simulink model "dcmotor"  (R2023b)
settings: Solver=VariableStepAuto  StartTime=0.0  StopTime=10  RelTol=10e-6
undefined symbols (not defined in the file): B, J, Ke, Ki, Kp, Kt, La, Ra, TL
settings Model: Creator=FM22  LastModifiedBy=FM22

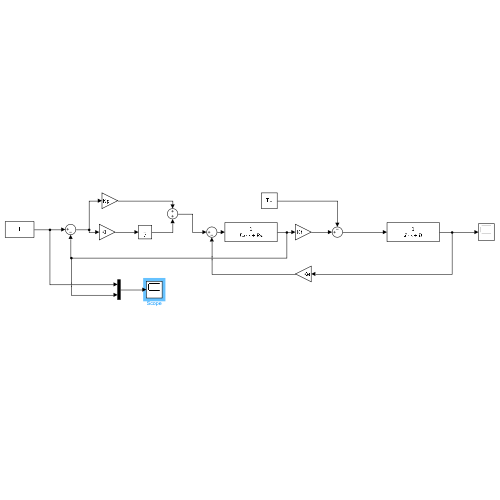
[thumbnail: Simulink's stored preview of the top-level diagram]
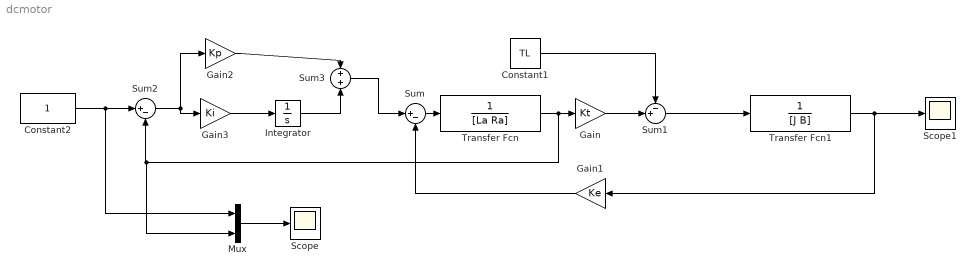
== system dcmotor ==
  Constant1 : Constant  Value=TL
  Constant2 : Constant
  Gain : Gain  Gain=Kt
  Gain1 : Gain  Gain=Ke
  Gain2 : Gain  Gain=Kp
  Gain3 : Gain  Gain=Ki
  Integrator : Integrator
  Mux : Mux  Inputs=2
  Scope : Scope
  Scope1 : Scope
  Sum : Sum  Inputs=|+-
  Sum1 : Sum  Inputs=-+|
  Sum2 : Sum  Inputs=|+-
  Sum3 : Sum  Inputs=+|+
  Transfer Fcn : TransferFcn  Denominator=[La Ra]
  Transfer Fcn1 : TransferFcn  Denominator=[J B]  ParameterTunability=Unconstrained
  wires:
  Sum/1 -> Transfer Fcn/1
  Transfer Fcn/1 -> Mux/2, Sum2/2, Gain/1
  Gain/1 -> Sum1/2
  Constant1/1 -> Sum1/1
  Sum1/1 -> Transfer Fcn1/1
  Gain1/1 -> Sum/2
  Transfer Fcn1/1 -> Scope1/1, Gain1/1
  Constant2/1 -> Mux/1, Sum2/1
  Sum2/1 -> Gain2/1, Gain3/1
  Gain3/1 -> Integrator/1
  Integrator/1 -> Sum3/2
  Gain2/1 -> Sum3/1
  Sum3/1 -> Sum/1
  Mux/1 -> Scope/1
